simulink model "state_space_model"  (R2022b)
settings: Solver=VariableStepAuto  StartTime=0.0  StopTime=5  RelTol=1e-3
undefined symbols (not defined in the file): A_hat, b_hat, DiscIntNeverNeededParam, F_new, init_cond, Ts
settings Model: Creator=ninj2  LastModifiedBy=ninj2
settings DebuggingCC: UnconnectedInputMsg=warning  UnconnectedOutputMsg=warning  UnconnectedLineMsg=warning
settings ModelReferenceCC: EnableRefExpFcnMdlSchedulingChecks=on
settings RTWCC: DLArmComputeVersion=19.05

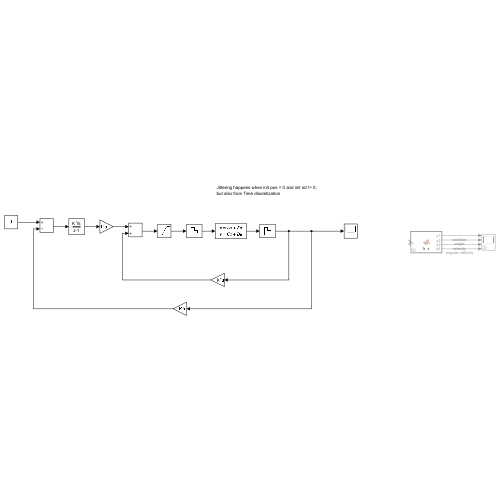
[thumbnail: Simulink's stored preview of the top-level diagram]
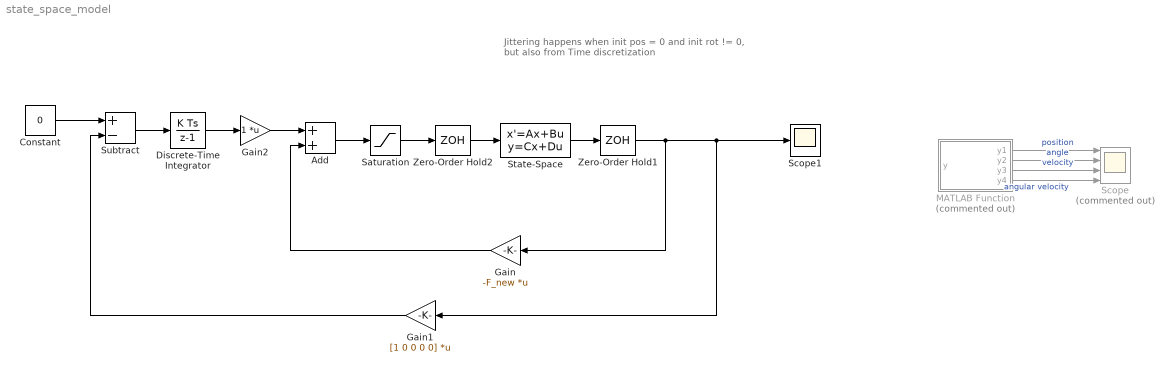
== system state_space_model ==
  note: Jittering happens when init pos = 0 and init rot != 0,
      | but also from Time discretization
  Add : Sum
  Constant : Constant  Value=0
  Discrete-Time Integrator : DiscreteIntegrator  SampleTime=-1  ICPrevOutput=DiscIntNeverNeededParam  ICPrevScaledInput=DiscIntNeverNeededParam
  Gain : Gain  Gain=-F_new  Multiplication=Matrix(K*u)
  Gain1 : Gain  Gain=[1 0 0 0 0]  Multiplication=Matrix(K*u)
  Gain2 : Gain  Multiplication=Matrix(K*u)
  MATLAB Function : MATLAB Function  Commented=on  TreatAsAtomicUnit=on
  Saturation : Saturate  UpperLimit=9  LowerLimit=-9  LinearizeAsGain=off
  Scope : Scope  Commented=on  NumInputPorts=4
  Scope1 : Scope
  State-Space : StateSpace  A=A_hat  B=b_hat  C=eye(5)  D=[0; 0; 0; 0; 0]  InitialCondition=[init_cond, 0]
  Subtract : Sum  Inputs=+-
  Zero-Order Hold1 : ZeroOrderHold  SampleTime=Ts
  Zero-Order Hold2 : ZeroOrderHold  SampleTime=Ts
  wires:
  MATLAB Function/1(y1) -> Scope/1  "position"
  MATLAB Function/2(y2) -> Scope/2  "angle"
  MATLAB Function/3(y3) -> Scope/3  "velocity"
  MATLAB Function/4(y4) -> Scope/4  "angular velocity"
  State-Space/1 -> Zero-Order Hold1/1
  Zero-Order Hold1/1 -> Gain/1, Gain1/1, Scope1/1
  Gain/1 -> Add/2
  Saturation/1 -> Zero-Order Hold2/1
  Zero-Order Hold2/1 -> State-Space/1
  Discrete-Time Integrator/1 -> Gain2/1
  Subtract/1 -> Discrete-Time Integrator/1
  Constant/1 -> Subtract/1
  Gain1/1 -> Subtract/2
  Gain2/1 -> Add/1
  Add/1 -> Saturation/1

== matlab function state_space_model/MATLAB Function ==
  data: y input; y1 output; y2 output; y3 output; y4 output
function [y1, y2, y3, y4]= fcn(y)

y1 = y(1);
y2 = y(2);
y3 = y(3);
y4 = y(4);
